simulink model "sim"  (R2016a)
settings: Solver=VariableStepAuto  StartTime=0.0  StopTime=20  RelTol=1e-3
libraries: fuzblock x1
settings Model: Creator=SPDKH  LastModifiedBy=SPDKH

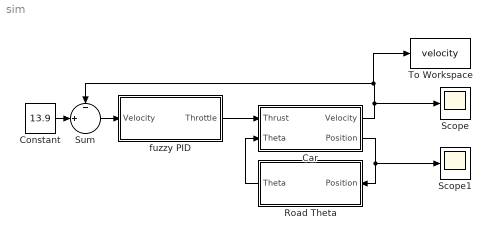
== system sim ==
  Car : Subsystem
  Constant : Constant  Value=13.9
  Road Theta : Subsystem
  Scope : Scope
  Scope1 : Scope
  Sum : Sum  Inputs=-|+||
  To Workspace : ToWorkspace  VariableName=velocity  SaveFormat=Timeseries  SampleTime=-1
  "fuzzy PID " : Subsystem
  wires:
  "fuzzy PID "/1(Throttle) -> Car/1(Thrust)
  Road Theta/1(Theta) -> Car/2(Theta)
  Car/2(Position) -> Scope1/1, Road Theta/1(Position)
  Sum/1 -> "fuzzy PID "/1(Velocity)
  Car/1(Velocity) -> Scope/1, To Workspace/1, Sum/1
  Constant/1 -> Sum/2

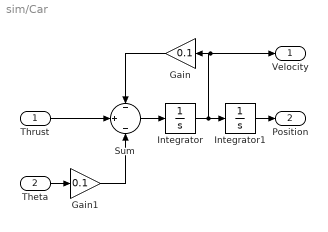
== system sim/Car ==
  Thrust : Inport
  Theta : Inport  Port=2
  Gain : Gain  Gain=0.1
  Gain1 : Gain  Gain=0.1
  Integrator : Integrator
  Integrator1 : Integrator
  Sum : Sum  Inputs=-|+|-
  Velocity : Outport
  Position : Outport  Port=2
  wires:
  Sum/1 -> Integrator/1
  Integrator/1 -> Velocity/1, Gain/1, Integrator1/1
  Gain/1 -> Sum/1
  Theta/1 -> Gain1/1
  Gain1/1 -> Sum/3
  Thrust/1 -> Sum/2
  Integrator1/1 -> Position/1

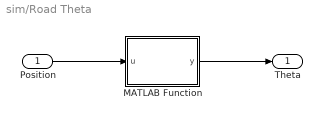
== system sim/Road Theta ==
  Position : Inport
  MATLAB Function : MATLAB Function  TreatAsAtomicUnit=on
  Theta : Outport
  wires:
  Position/1 -> MATLAB Function/1(u)
  MATLAB Function/1(y) -> Theta/1

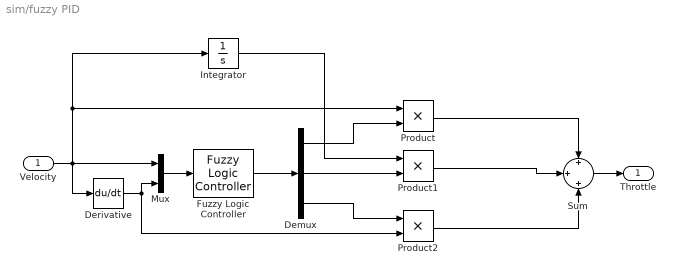
== system sim/fuzzy PID  ==
  Velocity : Inport
  Demux : Demux  Outputs=3
  Derivative : Derivative
  Fuzzy Logic Controller : fuzblock/Fuzzy Logic  Controller  fis=['Rules.fis']
  Integrator : Integrator
  Mux : Mux  Inputs=2
  Product : Product
  Product1 : Product
  Product2 : Product
  Sum : Sum  Inputs=+|+|+
  Throttle : Outport
  wires:
  Sum/1 -> Throttle/1
  Fuzzy Logic Controller/1 -> Demux/1
  Demux/2 -> Product1/2
  Demux/1 -> Product/2
  Demux/3 -> Product2/1
  Mux/1 -> Fuzzy Logic Controller/1
  Velocity/1 -> Integrator/1, Product/1, Derivative/1, Mux/1
  Derivative/1 -> Product2/2, Mux/2
  Integrator/1 -> Product1/1
  Product1/1 -> Sum/2
  Product/1 -> Sum/1
  Product2/1 -> Sum/3

== matlab function sim/Road Theta/MATLAB Function ==
  data: u input; y output
function y = fcn(u)

	if u < 0 
        y = -5;
    elseif u < 20 
        y = -5 + u/4;
    elseif u < 40
        y = 0;
    elseif u < 80
        y = -10 + u/4;
    else
        y = 10;
    end
    
end
